simulink model "kalman_filter"  (R2018a)
settings: Solver=FixedStepDiscrete  StartTime=0.0  StopTime=10.0  RelTol=1e-3
model workspace (MAT data in the model file):
  P0 = Simulink.Parameter
  P0.Value = [1  0  0  0  0  0; 0  1  0  0  0  0; 0  0  1  0  0  0; 0  0  0  1  0  0; 0  0  0  0  1  0; 0  0  0  0  0  1]
  P0.DataType = 'auto'
  P0.Dimensions = [6 6]
  Q = Simulink.Parameter
  Q.Value = [1  0  0  0  0  0; 0  1  0  0  0  0; 0  0  1  0  0  0; 0  0  0  1  0  0; 0  0  0  0  1  0; 0  0  0  0  0  1]
  Q.DataType = 'auto'
  Q.Dimensions = [6 6]
  R = Simulink.Parameter
  R.Value = [1  0  0  0  0  0; 0  1  0  0  0  0; 0  0  1  0  0  0; 0  0  0  1  0  0; 0  0  0  0  1  0; 0  0  0  0  0  1]
  R.DataType = 'auto'
  R.Dimensions = [6 6]
  dt = Simulink.Parameter
  dt.Value = 0.02
  dt.DataType = 'double'
  dt.Dimensions = [1 1]
  x0 = Simulink.Parameter
  x0.Value = [0; 0; 0; 0; 0; 0]
  x0.DataType = 'auto'
  x0.Dimensions = [6 1]
settings Model: ParameterArgumentNames=dt  OrderedModelArguments=off  Creator=Test  LastModifiedBy=Test

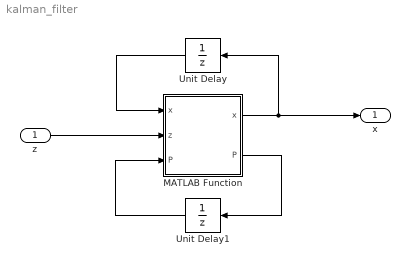
== system kalman_filter ==
  z : Inport
  MATLAB Function : MATLAB Function  TreatAsAtomicUnit=on  mask{Q=0, R=0, dt=dt}
      mask prompts: dt "Sample Time"
  Unit Delay : UnitDelay  InitialCondition=x0  SampleTime=-1
  Unit Delay1 : UnitDelay  InitialCondition=P0  SampleTime=-1
  x : Outport
  wires:
  MATLAB Function/1(x) -> Unit Delay/1, x/1
  Unit Delay/1 -> MATLAB Function/1("x ")
  z/1 -> MATLAB Function/2(z)
  MATLAB Function/2(P) -> Unit Delay1/1
  Unit Delay1/1 -> MATLAB Function/3("P ")

== matlab function kalman_filter/MATLAB Function ==
  data: x input; z input; x output; P output; P input; Q parameter; R parameter; dt parameter
function [x, P] = ekf(x, z, P, Q, R, dt)

[x, P] = predict(x, P, Q, dt);
[x, P] = update(z, x, P, R);

end

function [x, P] = predict(x, P, Q, dt)
% [x, P] = predict(x, P, Q, dt)
%
% predict states and covariance

phi = x(4);
theta = x(5);
psi = x(6);

R_e2b = [
    1 sin(phi)*tan(theta) cos(phi)*tan(theta);
    0 cos(phi) -sin(phi);
    0 sin(phi)/cos(theta) cos(phi)/cos(theta)];
M = [eye(3,3) zeros(3,3);
    R_e2b*dt, eye(3,3)];
x = M*x;

F = Fj(x, dt);
P = F*P*F'+Q;

end

function [x, P] = update(z, x, P, R)

p = x(1);
q = x(2);
r = x(3);
phi = x(4);
theta = x(5);
psi = x(6);

g = 9.81;
z1_est = [p, q, r];
z2_est = g*[-sin(theta), sin(phi)*cos(theta), cos(phi)*cos(theta)];
z_est = [z1_est, z2_est]';
y = z - z_est;

H = Hj(x);
S = H*P*H'+R;
K = P*H'*inv(S);

nr = size(K,1);
nc = size(H,1);
x = x + K*y;
P = (eye(nr,nc)-K*H)*P;

end

function mat = Fj(x, dt)
p = x(1);
q = x(2);
r = x(3);
phi = x(4);
theta = x(5);
psi = x(6);

% To-Do: compute Jacobian
J1 = [
    1 sin(phi)*tan(theta) cos(phi)*tan(theta);
    0 cos(phi) -sin(phi);
    0 sin(phi)/cos(theta) cos(phi)/cos(theta)];

% To-Do: compute Jacobian
J2 = zeros(3,3);
mat = [eye(3,3), zeros(3,3);
    J1*dt, J2];

end


function mat = Hj(x)
p = x(1);
q = x(2);
r = x(3);
phi = x(4);
theta = x(5);
psi = x(6);

g = 9.81;
J = zeros(3,3);
J(1,2) = -g*cos(theta);
J(2,1) = g*(cos(phi)*cos(theta));
J(2,2) = g*(-sin(phi)*sin(theta));
J(3,1) = g*(-sin(phi)*cos(theta));
J(3,2) = g*(-cos(phi)*sin(theta));
mat = [eye(3,3), zeros(3,3);
    zeros(3,3), J];
end
